simulink library "Pump_Additional"  (Simulink 8.2)
settings: Solver=ode45  StartTime=0.0  StopTime=10.0  RelTol=1e-3
undefined symbols (not defined in the file): DiameterLastPiece, DPConstant, DPLinear, DPQuadratic, ID, Pressure, Temperature
libraries: carnot x3
settings Model: Creator=lena.frank  LastModifiedBy=drhf

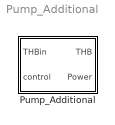
== system Pump_Additional ==
  Pump_Additional : Subsystem  mask(additional pump){a0=2.0e4, a1=-7000, a2=0 %-3e-3, dia=0.025, t1=5, ua=0, mcp=0, tamb=0}
      mask prompts: a0 "pump characteristic: constant coefficient [Pa]"; a1 "pump characteristic: linear coefficient [Pa*s/kg]"; a2 "pump characteristic: quadratic coefficient [Pa*(s/kg)²]"; dia "diameter at in- and outlet [m]"; t1 "time constant in s"; ua "losses to ambient  in W/K"; mcp "thermal capacity in J/K"; tamb "ambient temperatature in °C"
      mask help: This pump is an additional pump in a circuit. Every circuit must have exactly ONE 'pump_main'. It may have several 'pump_additional' blocks.
      mask init:
      | t=1;
      mask Help: web(fullfile(path_carnot('help'),'Pump_Main.html'),'-helpbrowser')
      mask Display:
      | plot(0,0,100,100,[40,70,40,30,30,40,60,70,70,60,40],[70,50,30,40,60,70,70,60,40,30,30])
      | port_label('input',1,'THB')
      | port_label('input',2,'ctr')
      | port_label('output',1,'THB')
      | port_label('output',2,'Pel')

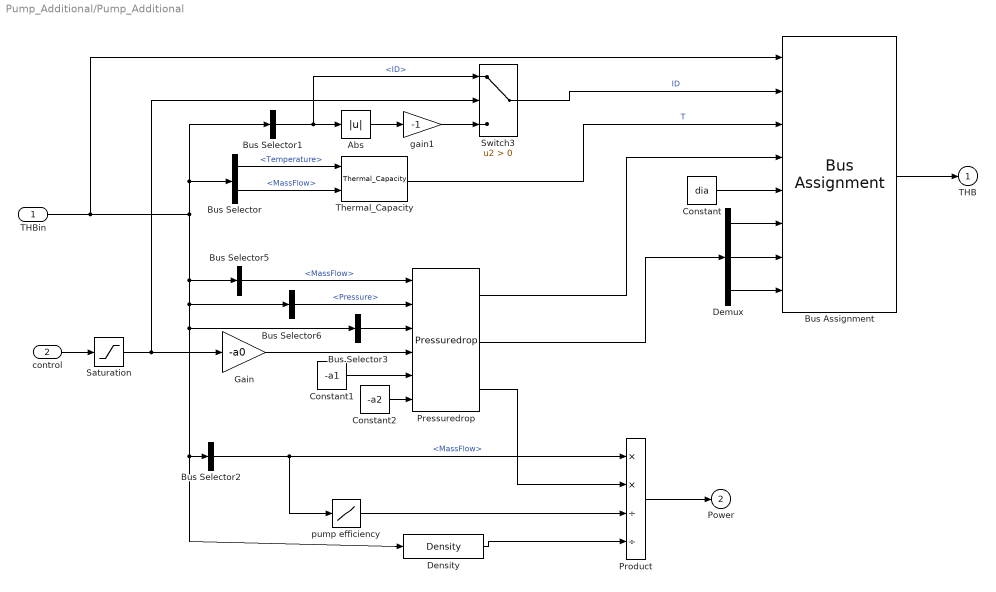
== system Pump_Additional/Pump_Additional ==
  THBin : Inport
  control : Inport  Port=2
  Abs : Abs
  Bus Assignment : BusAssignment  AssignedSignals=ID,Temperature,Pressure,DiameterLastPiece,DPConstant,DPLinear,DPQuadratic
  Bus Selector : BusSelector  OutputSignals=Temperature,MassFlow
  Bus Selector1 : BusSelector  OutputSignals=ID
  Bus Selector2 : BusSelector  OutputSignals=MassFlow
  Bus Selector3 : BusSelector  OutputSignals=DPConstant,DPLinear,DPQuadratic  OutputAsBus=on
  Bus Selector5 : BusSelector  OutputSignals=MassFlow
  Bus Selector6 : BusSelector  OutputSignals=Pressure
  Constant : Constant  Value=dia
  Constant1 : Constant  Value=-a1
  Constant2 : Constant  Value=-a2
  Demux : Demux  Outputs=3
  Density : carnot/Basic/Material_Properties/Density  VariantControl=CarlibClassic  INPUTARGUMENTS=THB  DEBUGLEVEL=DEBUGLEVEL  MAXTOTALWARNINGS=inf  MAXCONSECUTIVEWARNINGS=inf  WRITETOFILE=0  FILENAME='errors.txt'
  Gain : Gain  Gain=-a0
  Pressuredrop : carnot/Basic/Pressure_Drop/Pressuredrop
  Product : Product  Inputs=**//  SaturateOnIntegerOverflow=on  InputSameDT=on  OutDataTypeStr=Inherit: Same as first input
  Saturation : Saturate  UpperLimit=1  LowerLimit=0
  Switch3 : Switch  Criteria=u2 > Threshold  SaturateOnIntegerOverflow=on  InputSameDT=on
  Thermal_Capacity : carnot/Basic/Thermal_Models/Thermal_Capacity  UA=1  mcp=t1*100  Tamb=20
  gain1 : Gain  Gain=-1  SaturateOnIntegerOverflow=on  OutDataTypeStr=Inherit: Same as input  ParamDataTypeStr=Inherit: Same as input
  pump efficiency : Lookup  InputValues=0:1:5  Table=[0.001 0.5 0.7 0.7 0.5 0.001]  SaturateOnIntegerOverflow=on
  THB : Outport
  Power : Outport  Port=2
  wires:
  Thermal_Capacity/1 -> Bus Assignment/3  "T"
  control/1 -> Saturation/1
  Density/1 -> Product/4
  pump efficiency/1 -> Product/3
  THBin/1 -> Bus Selector/1, Bus Selector1/1, Bus Selector5/1, Bus Selector6/1, Bus Selector3/1, Density/1, Bus Selector2/1, Bus Assignment/1
  Product/1 -> Power/1
  Bus Selector/1 -> Thermal_Capacity/1  "<Temperature>"
  Bus Selector/2 -> Thermal_Capacity/2  "<MassFlow>"
  Bus Selector2/1 -> Product/1, pump efficiency/1  "<MassFlow>"
  Saturation/1 -> Switch3/2, Gain/1
  Bus Selector1/1 -> Switch3/1, Abs/1  "<ID>"
  Abs/1 -> gain1/1
  gain1/1 -> Switch3/3
  Switch3/1 -> Bus Assignment/2  "ID"
  Pressuredrop/3 -> Product/2
  Bus Selector5/1 -> Pressuredrop/1  "<MassFlow>"
  Bus Selector6/1 -> Pressuredrop/2  "<Pressure>"
  Bus Assignment/1 -> THB/1
  Pressuredrop/1 -> Bus Assignment/4
  Constant/1 -> Bus Assignment/5
  Bus Selector3/1 -> Pressuredrop/3
  Gain/1 -> Pressuredrop/4
  Constant1/1 -> Pressuredrop/5
  Constant2/1 -> Pressuredrop/6
  Pressuredrop/2 -> Demux/1
  Demux/1 -> Bus Assignment/6
  Demux/2 -> Bus Assignment/7
  Demux/3 -> Bus Assignment/8
